simulink model "multi_motor_encoder_Test"  (R2021b)
settings: Solver=FixedStepAuto  StartTime=0.0  StopTime=300  FixedStep=0.005  RelTol=1e-3  EnableMultiTasking=on
settings Model: Creator=The MathWorks, Inc.  LastModifiedBy=kboxi
settings SolverCC: AlgebraicLoopSolver=TrustRegion  PositivePriorityOrder=on
settings OptimizationCC: EnhancedBackFolding=on  PassReuseOutputArgsThreshold=0  MaxStackSize=64  OptimizeBlockOrder=speed  DifferentSizesBufferReuse=on  OptimizationCustomize=off
settings DebuggingCC: ParameterTunabilityLossMsg=error  SFMachineParentedDataDiag=warning
settings HardwareCC: ProdBitPerPointer=32  ProdBitPerSizeT=32  ProdBitPerPtrDiffT=32  ProdLargestAtomicInteger=Long  ProdLargestAtomicFloat=Double  ProdWordSize=32  ProdLongLongMode=on  ProdHWDeviceType=ARM Compatible->ARM Cortex  UseEmbeddedCoderFeatures=off
settings RTWCC: Description=Embedded Coder  SystemTargetFile=ert.tlc  HardwareBoard=Raspberry Pi  TLCOptions="-aInlineSetEventsForThisBaseRateFcn=TLC_FALSE -aSuppressMultiTaskScheduler=TLC_FALSE  -aRateBasedStepFcn=0"  TemplateMakefile=ert_default_tmf  Toolchain=GNU GCC Embedded Linux  BuildConfiguration=Faster Runs
settings CodeAppCC: ForceParamTrailComments=on  OperatorAnnotations=on
settings ERTTargetCC: ERTCustomFileBanners=off  SupportContinuousTime=on  SupportNonInlinedSFcns=on  RemoveResetFunc=off  SupportVariableSizeSignals=on  ModelStepFunctionPrototypeControlCompliant=off  ExtModeTransport=2  ExtModeStaticAlloc=on  ExtModeMexFile=ext_xcp  ExtModeIntrfLevel=Level2 - Open

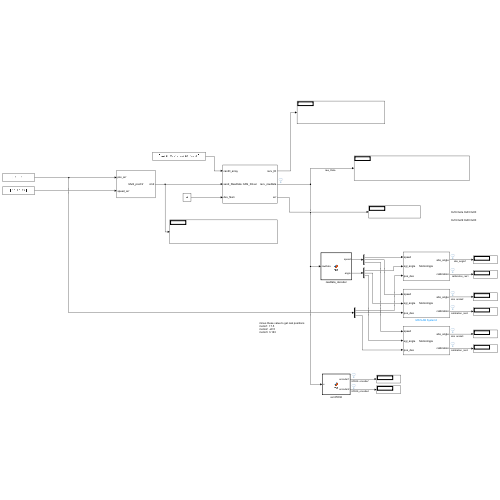
[thumbnail: Simulink's stored preview of the top-level diagram]
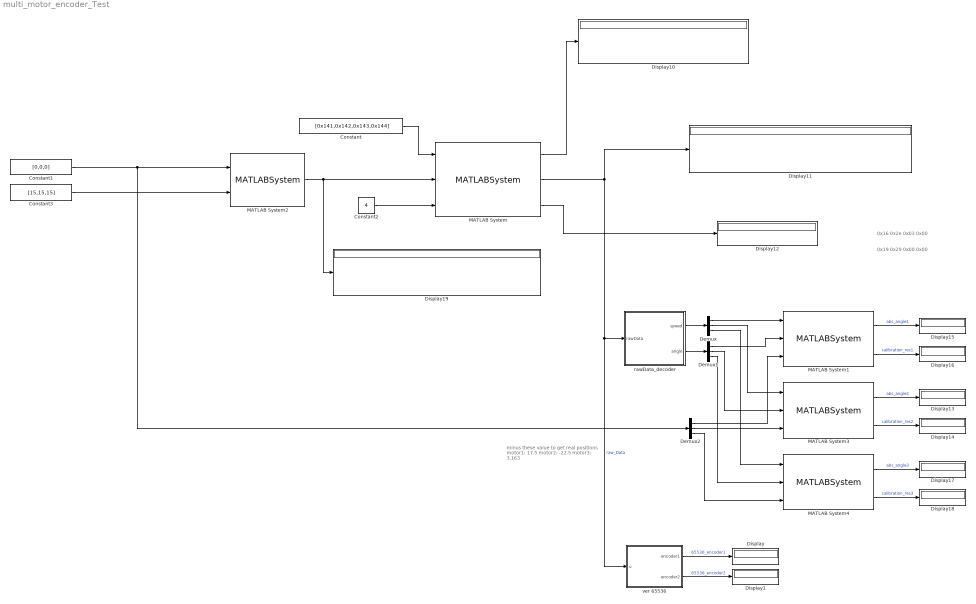
== system multi_motor_encoder_Test ==
  note: minus these value to get real positions
      | motor1: 17.5
      | motor2: -22.5
      | motor3: 3.163
  note: 0x19 0x29 0x00 0x00
  note: 0x16 0x2e 0x03 0x00
  Constant : Constant  Value=[0x141,0x142,0x143,0x144]
  Constant1 : Constant  Value=[0,0,0]
  Constant2 : Constant  Value=4  OutDataTypeStr=int32
  Constant3 : Constant  Value=[15,15,15]
  Demux : Demux  Outputs=3
  Demux1 : Demux  Outputs=3
  Demux2 : Demux  Outputs=3
  Display{,1,10..19} (12 alike) : Display
      Display10 settings: Format=hex (Stored Integer)
      Display11 settings: Format=hex (Stored Integer)
      Display12 settings: Format=hex (Stored Integer)
      Display19 settings: Format=hex (Stored Integer)
  MATLAB System : MATLABSystem  System=canSendRecv  canPort=can1
      mask Type: canSendRecv
      mask Display:
      | disp('CAN_Driver');
      | port_label('input',1,'canID_array');
      | port_label('input',2,'send_RawData');
      | port_label('input',3,'dev_Num');
      | port_label('output',1,'recv_ID');
      | port_label('output',2,'recv_rawData');
      | port_label('output',3,'err');
  MATLAB System1 : MATLABSystem  System=MotorAngle  angleOff=-17.5  SimulateUsing=Code generation
      mask Type: MotorAngle
      mask Display:
      | disp('MotorAngle');
      | port_label('input',1,'speed');
      | port_label('input',2,'sgl_angle');
      | port_label('input',3,'pos_des');
      | port_label('output',1,'abs_angle');
      | port_label('output',2,'calibration');
  MATLAB System2 : MATLABSystem  System=Multi_posCtr  SimulateUsing=Code generation
      mask Type: Multi_posCtr
      mask Display:
      | disp('Multi_posCtr');
      | port_label('input',1,'pos_arr');
      | port_label('input',2,'speed_arr');
      | port_label('output',1,'cmd');
  MATLAB System3 : MATLABSystem  System=MotorAngle  angleOff=22.5  SimulateUsing=Code generation
      mask Type: MotorAngle
      mask Display:
      | disp('MotorAngle');
      | port_label('input',1,'speed');
      | port_label('input',2,'sgl_angle');
      | port_label('input',3,'pos_des');
      | port_label('output',1,'abs_angle');
      | port_label('output',2,'calibration');
  MATLAB System4 : MATLABSystem  System=MotorAngle  angleOff=-3.163  SimulateUsing=Code generation
      mask Type: MotorAngle
      mask Display:
      | disp('MotorAngle');
      | port_label('input',1,'speed');
      | port_label('input',2,'sgl_angle');
      | port_label('input',3,'pos_des');
      | port_label('output',1,'abs_angle');
      | port_label('output',2,'calibration');
  rawData_decoder : MATLAB Function  TreatAsAtomicUnit=on
  ver 65536 : MATLAB Function  TreatAsAtomicUnit=on
  wires:
  Constant/1 -> MATLAB System/1
  MATLAB System2/1 -> Display19/1, MATLAB System/2
  Constant2/1 -> MATLAB System/3
  MATLAB System/1 -> Display10/1
  MATLAB System/2 -> Display11/1, ver 65536/1(u), rawData_decoder/1(rawData)  "raw_Data"
  MATLAB System/3 -> Display12/1
  Constant3/1 -> MATLAB System2/2
  Constant1/1 -> Demux2/1, MATLAB System2/1
  MATLAB System1/1 -> Display15/1  "abs_angle1"
  MATLAB System1/2 -> Display16/1  "calibration_res1"
  MATLAB System4/2 -> Display18/1  "calibration_res3"
  MATLAB System4/1 -> Display17/1  "abs_angle3"
  MATLAB System3/2 -> Display14/1  "calibration_res2"
  MATLAB System3/1 -> Display13/1  "abs_angle2"
  rawData_decoder/2(angle) -> Demux1/1
  rawData_decoder/1(speed) -> Demux/1
  Demux/1 -> MATLAB System1/1
  Demux/2 -> MATLAB System3/1
  Demux/3 -> MATLAB System4/1
  Demux1/1 -> MATLAB System1/2
  Demux1/2 -> MATLAB System3/2
  Demux1/3 -> MATLAB System4/2
  Demux2/1 -> MATLAB System1/3
  Demux2/2 -> MATLAB System3/3
  Demux2/3 -> MATLAB System4/3
  ver 65536/1(encoder1) -> Display/1  "65536_encoder1"
  ver 65536/2(encoder2) -> Display1/1  "65536_encoder2"

== matlab function multi_motor_encoder_Test/rawData_decoder ==
  data: speed output; rawData input uint8; angle output
function [speed,angle] = fcn(rawData)
% angle : single loop position, degree
% speed : speed after the reducer, degree per second
angle=zeros(3,1);
speed=zeros(3,1);
for i=1:1:3
    idx=i*8-7;
    angle(i) = double(typecast(rawData(idx+6:idx+7),'uint16'))/65535*360;
    speed(i) = double(typecast(rawData(idx+4:idx+5),'int16'))/6;
end

== matlab function multi_motor_encoder_Test/ver 65536 ==
  data: u input uint8; encoder1 output; encoder2 output
function [encoder1,encoder2] = fcn(u)
rowEnd=u(25:32);
encoder1=double(typecast(rowEnd(1:2),'uint16'))/65536*360;
encoder2=double(typecast(rowEnd(3:4),'uint16'))/65536*360;
